simulink model "PendelModel_SingularError_SIM"  (R2017b)
settings: Solver=FixedStepAuto  StartTime=0.0  StopTime=100.0  FixedStep=0.001  RelTol=1e-3
values from neighbouring files (symbols this model uses):
  K1 = (g * mK*l_AC+mR*l_AB)/IK    (= 35.6940657896)    [ParameterInit.m]
  K2 = (Cphi + Cpsi)/IK    (= 1.13375244539)    [ParameterInit.m]
  K3 = Cpsi/IK    (= 0.00567242302855)    [ParameterInit.m]
  K4 = 1/IK    (= 181.948390703)    [ParameterInit.m]
  K5 = Cpsi/IR    (= 0.266849268167)    [ParameterInit.m]
  K6 = 1/IR    (= 8559.44534794)    [ParameterInit.m]
  phi_0 = phi(1)    [ParameterInit.m]
  uK_0 = uk(1)    [ParameterInit.m]
  uR_0 = ur(1)    [ParameterInit.m]
undefined symbols (not defined in the file or in its folder): magnitude
settings Model: Creator=michael  LastModifiedBy=michael

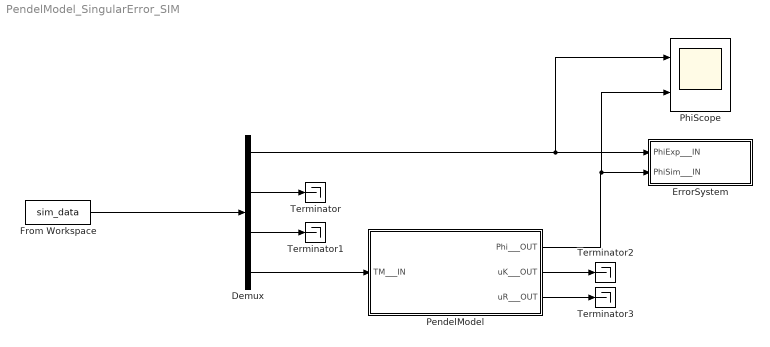
== system PendelModel_SingularError_SIM ==
  Demux : Demux
  ErrorSystem : Subsystem
  From Workspace : FromWorkspace  VariableName=sim_data  SampleTime=0
  PendelModel : Subsystem
  PhiScope : Scope  NumInputPorts=2
  Terminator{,1..3} (4 alike) : Terminator
  wires:
  PendelModel/1(Phi___OUT) -> PhiScope/2, ErrorSystem/2(PhiSim___IN)
  From Workspace/1 -> Demux/1
  Demux/4 -> PendelModel/1(TM___IN)
  Demux/2 -> Terminator/1
  Demux/3 -> Terminator1/1
  Demux/1 -> PhiScope/1, ErrorSystem/1(PhiExp___IN)
  PendelModel/2(uK___OUT) -> Terminator2/1
  PendelModel/3(uR___OUT) -> Terminator3/1

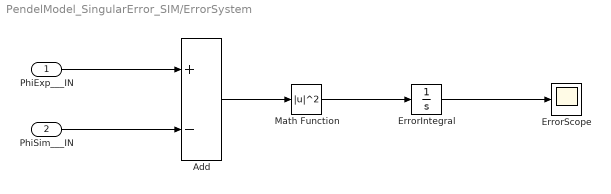
== system PendelModel_SingularError_SIM/ErrorSystem ==
  PhiExp___IN : Inport
  PhiSim___IN : Inport  Port=2
  Add : Sum  Inputs=+-
  ErrorIntegral : Integrator
  ErrorScope : Scope
  Math Function : Math  Operator=magnitude^2  SaturateOnIntegerOverflow=on
  wires:
  PhiExp___IN/1 -> Add/1
  PhiSim___IN/1 -> Add/2
  ErrorIntegral/1 -> ErrorScope/1
  Add/1 -> Math Function/1
  Math Function/1 -> ErrorIntegral/1

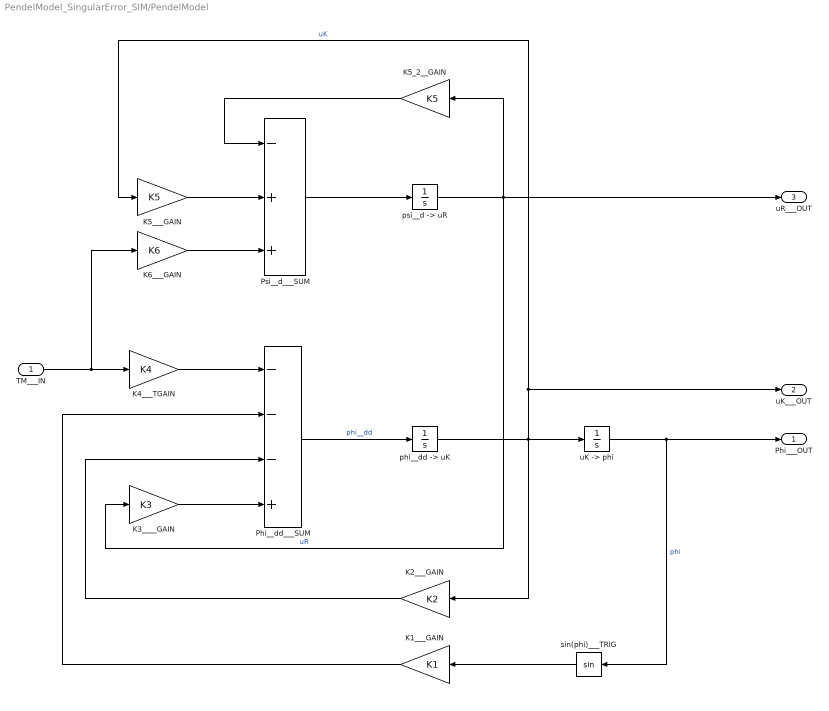
== system PendelModel_SingularError_SIM/PendelModel ==
  TM___IN : Inport
  K1___GAIN : Gain  Gain=K1
  K2___GAIN : Gain  Gain=K2
  K3____GAIN : Gain  Gain=K3
  K4___TGAIN : Gain  Gain=K4
  K5_2__GAIN : Gain  Gain=K5
  K5___GAIN : Gain  Gain=K5
  K6___GAIN : Gain  Gain=K6
  Phi__dd___SUM : Sum  Inputs=---+
  Psi__d___SUM : Sum  Inputs=-++
  "phi__dd -> uK" : Integrator  InitialCondition=uK_0
  "psi__d -> uR" : Integrator  InitialCondition=uR_0
  sin(phi)___TRIG : Trigonometry
  "uK -> phi" : Integrator  InitialCondition=phi_0
  Phi___OUT : Outport
  uK___OUT : Outport  Port=2
  uR___OUT : Outport  Port=3
  wires:
  TM___IN/1 -> K6___GAIN/1, K4___TGAIN/1
  K4___TGAIN/1 -> Phi__dd___SUM/1
  Phi__dd___SUM/1 -> "phi__dd -> uK"/1  "phi__dd"
  "phi__dd -> uK"/1 -> K2___GAIN/1, uK___OUT/1, K5___GAIN/1, "uK -> phi"/1  "uK"
  "uK -> phi"/1 -> Phi___OUT/1, sin(phi)___TRIG/1  "phi"
  sin(phi)___TRIG/1 -> K1___GAIN/1
  K1___GAIN/1 -> Phi__dd___SUM/2
  K2___GAIN/1 -> Phi__dd___SUM/3
  K6___GAIN/1 -> Psi__d___SUM/3
  K5___GAIN/1 -> Psi__d___SUM/2
  Psi__d___SUM/1 -> "psi__d -> uR"/1
  "psi__d -> uR"/1 -> K3____GAIN/1, uR___OUT/1, K5_2__GAIN/1  "uR"
  K5_2__GAIN/1 -> Psi__d___SUM/1
  K3____GAIN/1 -> Phi__dd___SUM/4
